simulink model "MODEL_SS"  (R2024b)
settings: Solver=VariableStepAuto  StartTime=0.0  StopTime=25  RelTol=1e-3
undefined symbols (not defined in the file or in its folder): A, B
settings Model: Creator=amrmo  LastModifiedBy=amrmo

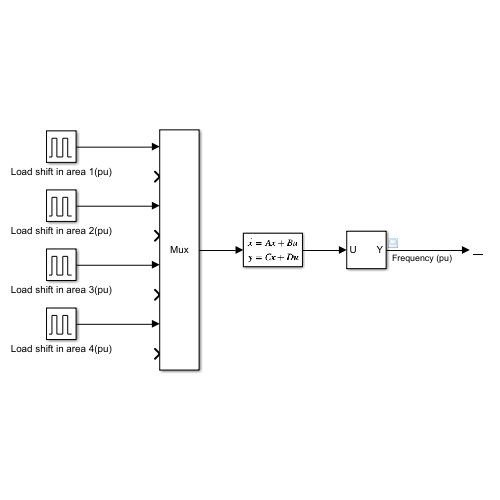
[thumbnail: Simulink's stored preview of the top-level diagram]
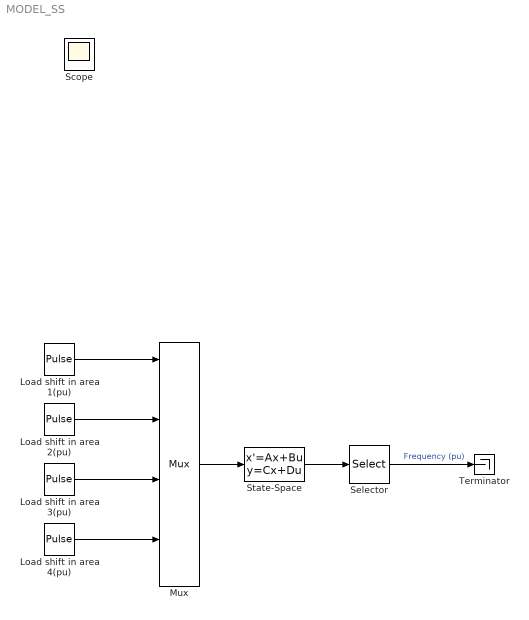
== system MODEL_SS ==
  Load shift in area 1(pu) : DiscretePulseGenerator  PulseType=Time based  Amplitude=0.1  Period=10  PulseWidth=5
  Load shift in area 2(pu) : DiscretePulseGenerator  PulseType=Time based  Amplitude=0  Period=10  PulseWidth=5
  Load shift in area 3(pu) : DiscretePulseGenerator  PulseType=Time based  Amplitude=0  Period=10  PulseWidth=5
  Load shift in area 4(pu) : DiscretePulseGenerator  PulseType=Time based  Amplitude=0  Period=10  PulseWidth=5
  Mux : Mux  Inputs=8
  Selector : Selector  InputPortWidth=16  IndexOptions=Index vector (dialog)  Indices=[3, 7, 11, 15]  OutputSizes=1
  State-Space : StateSpace  A=A  B=B  C=eye(size(A,1))  D=zeros(size(A,1), size(B,2))  InitialCondition=0
  Terminator : Terminator
  Scope : Scope
  wires:
  Mux/1 -> State-Space/1
  Load shift in area 1(pu)/1 -> Mux/1
  Load shift in area 2(pu)/1 -> Mux/3
  Load shift in area 3(pu)/1 -> Mux/5
  Load shift in area 4(pu)/1 -> Mux/7
  State-Space/1 -> Selector/1
  Selector/1 -> Terminator/1  "Frequency (pu)"
